simulink model "sim_1_3"  (R2022b)
settings: Solver=VariableStepAuto  StartTime=0.0  StopTime=8  FixedStep=0.0001  MaxStep=0.001  RelTol=1e-3
values from neighbouring files (symbols this model uses):
  a_sin = [pi/2; pi/2; 0.2; pi/2]    [par_1_3.m]
  Kd = 1000*eye(4)    [par_1_3.m]
  Kp = 1000*eye(4)    [par_1_3.m]
  omega_sin = 10*[1; 1; 1; 1]    [par_1_3.m]
  q_0 = [pi/2;pi/4;0;0]    [par_1_3.m]
  q_dot_0 = [0;0;0;0]    [par_1_3.m]
undefined symbols (not defined in the file or in its folder): a_filt, b_filt
settings Model: Creator=Alberto  LastModifiedBy=david
settings SolverCC: MaxConsecutiveMinStep=100000  AlgebraicLoopSolver=TrustRegion
settings DebuggingCC: UnconnectedInputMsg=warning  UnconnectedOutputMsg=warning  UnconnectedLineMsg=warning  SFMachineParentedDataDiag=warning
settings ModelReferenceCC: EnableRefExpFcnMdlSchedulingChecks=on
settings RTWCC: DLArmComputeVersion=19.05

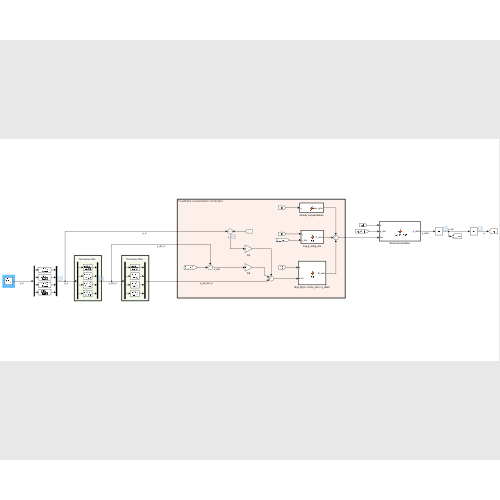
[thumbnail: Simulink's stored preview of the top-level diagram]
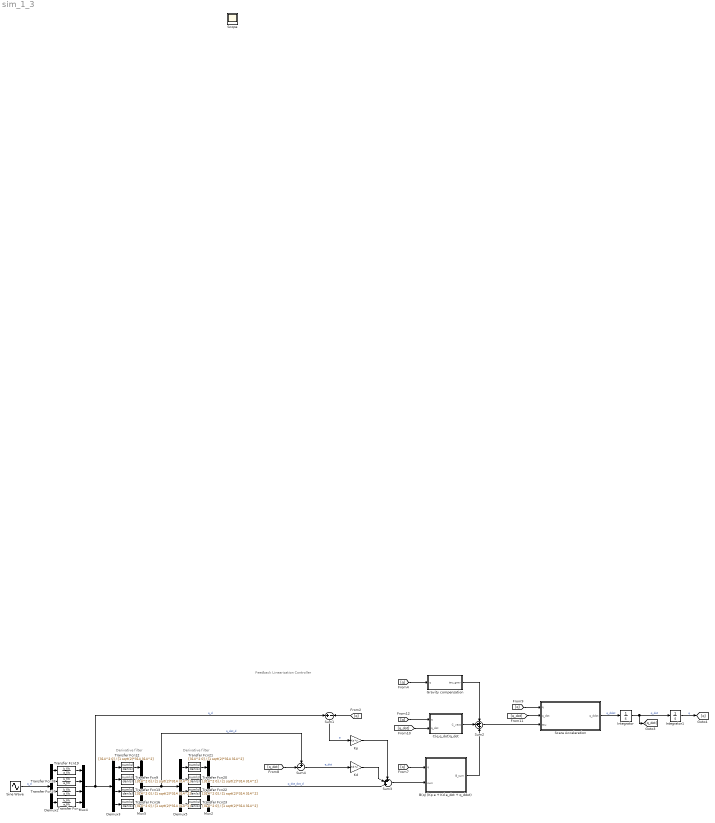
== system sim_1_3 ==
  note: Feedback Linearization Controller
  note: Derivative filter
  note: Derivative filter
  B(q) (Kp e + Kd e_dot + q_ddot) : MATLAB Function  TreatAsAtomicUnit=on
  C(q,q_dot)q_dot : MATLAB Function  TreatAsAtomicUnit=on
  Demux2 : Demux
  Demux3 : Demux
  Demux5 : Demux
  Gravity compensation : MATLAB Function  TreatAsAtomicUnit=on
  Integrator : Integrator  InitialCondition=q_dot_0
  Integrator1 : Integrator  InitialCondition=q_0
  Kd : Gain  Gain=Kd  Multiplication=Matrix(K*u)
  Kp : Gain  Gain=Kp  Multiplication=Matrix(K*u)
  Mux2 : Mux
  Mux4 : Mux
  Mux5 : Mux
  Scara Acceleration : MATLAB Function  TreatAsAtomicUnit=on
  Sine Wave : Sin  Amplitude=a_sin  Frequency=omega_sin  SampleTime=0
  Sum1 : Sum  Inputs=+-
  Sum2 : Sum  Inputs=+++
  Sum3 : Sum  Inputs=+++|
  Sum4 : Sum  Inputs=+-|
  Transfer Fcn{,17..19} (4 alike) : TransferFcn  Numerator=b_filt  Denominator=a_filt
  Transfer Fcn{9,12..13,16,20..23} (8 alike) : TransferFcn  Numerator=[314^2 0]  Denominator=[1 sqrt(2)*314 314^2]
  Scope : Scope
  wires:
  Demux3/4 -> Transfer Fcn16/1
  Transfer Fcn12/1 -> Mux5/1
  Transfer Fcn16/1 -> Mux5/4
  Demux3/1 -> Transfer Fcn12/1
  Demux3/3 -> Transfer Fcn13/1
  Transfer Fcn/1 -> Mux4/4
  Integrator/1 -> [q_dot], Integrator1/1  "q_dot"
  Scara Acceleration/1(q_ddot) -> Integrator/1  "q_ddot"
  Demux3/2 -> Transfer Fcn9/1
  [q_dot] -> Scara Acceleration/2(q_dot)
  [q] -> Scara Acceleration/1(q)
  Mux4/1 -> Sum1/1, Demux3/1  "q_d"
  Transfer Fcn17/1 -> Mux4/3
  Transfer Fcn18/1 -> Mux4/2
  Transfer Fcn9/1 -> Mux5/2
  Integrator1/1 -> [q]  "q"
  Demux2/3 -> Transfer Fcn17/1
  Transfer Fcn13/1 -> Mux5/3
  Demux2/1 -> Transfer Fcn19/1
  Transfer Fcn19/1 -> Mux4/1
  Demux2/2 -> Transfer Fcn18/1
  Demux2/4 -> Transfer Fcn/1
  Sine Wave/1 -> Demux2/1  "q_d"
  Transfer Fcn22/1 -> Mux2/3
  Transfer Fcn20/1 -> Mux2/2
  Demux5/2 -> Transfer Fcn20/1
  Transfer Fcn21/1 -> Mux2/1
  Transfer Fcn23/1 -> Mux2/4
  Mux2/1 -> Sum3/3  "q_dot_dot_d"
  Demux5/3 -> Transfer Fcn22/1
  Demux5/1 -> Transfer Fcn21/1
  Demux5/4 -> Transfer Fcn23/1
  Sum4/1 -> Kd/1  "e_dot"
  Kp/1 -> Sum3/1
  [q_dot] -> C(q,q_dot)q_dot/2(q_dot)
  C(q,q_dot)q_dot/1(C_vect) -> Sum2/2
  [q] -> B(q) (Kp e + Kd e_dot + q_ddot)/1(q)
  [q] -> Gravity compensation/1(q)
  B(q) (Kp e + Kd e_dot + q_ddot)/1(B_sum) -> Sum2/3
  Sum1/1 -> Kp/1  "e"
  Gravity compensation/1(tau_grav) -> Sum2/1
  Sum3/1 -> B(q) (Kp e + Kd e_dot + q_ddot)/2(sum)
  [q_dot] -> Sum4/2
  Mux5/1 -> Sum4/1, Demux5/1  "q_dot_d"
  Kd/1 -> Sum3/2
  [q] -> Sum1/2
  [q] -> C(q,q_dot)q_dot/1(q)
  Sum2/1 -> Scara Acceleration/3(tau)

== matlab function sim_1_3/Scara Acceleration ==
  data: q input; q_ddot output; q_dot input; tau input
function q_ddot = SCARA_acc(q, q_dot, tau)%#codegen
coder.extrinsic('f_B_mex'); 
coder.extrinsic('f_C_vect_mex'); 
coder.extrinsic('f_g_vect_mex');
B = eye(4);
C_vect = zeros(4,1);
F_g = zeros(4,1);
tau = reshape(tau,4,1);
q_ddot = zeros(4,1);
B = full(f_B_mex('f_B',q));
C_vect = full(f_C_vect_mex('f_C_vect', q, q_dot));
F_g = full(f_g_vect_mex('f_g_vect', q));
q_ddot = (eye(4)/B)*(-C_vect-F_g+tau);

== matlab function sim_1_3/C(q,q_dot)q_dot ==
  data: q input; q_dot input; C_vect output
function C_vect = fcn(q, q_dot)%#codegen
coder.extrinsic('f_C_vect_mex'); 
C_vect = zeros(4,1);
C_vect = reshape(full(f_C_vect_mex('f_C_vect', q, q_dot)),4 ,1);

== matlab function sim_1_3/Gravity compensation ==
  data: q input; tau_grav output
function tau_grav = fcn(q)%#codegen
coder.extrinsic('f_g_vect_mex');
tau_grav = zeros(4,1);
tau_grav = reshape(full(f_g_vect_mex('f_g_vect', q)),4,1);

== matlab function sim_1_3/B(q) (Kp e + Kd e_dot + q_ddot) ==
  data: q input; B_sum output; sum input
function B_sum = fcn(q, sum)%#codegen
coder.extrinsic('f_B_mex'); 
B = eye(4);
B = full(f_B_mex('f_B',q));
B_sum = B * sum;
